simulink model "sistema_polo_polo"  (R2016a)
settings: Solver=ode45  SolverMode=SingleTasking  StartTime=0  StopTime=1.58  FixedStep=Ts_Power  RelTol=1e-3  AbsTol=1e-2
InitFcn:
  | Fnom = 50;        % Hz
  | 
  | Fc = 27*Fnom;   % (Hz)
  | Ts_Power = 1/(Fc*100);
  | Ts_Control = Ts_Power*10;
values from neighbouring files (symbols this model uses):
  L = 5    [obtencaodados.m]
undefined symbols (not defined in the file or in its folder): D1, Delta, DiscIntNeverNeededParam, magnitude
libraries: powerlib_meascontrol x56, powerlib x52
(part 4 of 4)

== system sistema_polo_polo/VSC Controller Station 2/Discrete VSC Controller /Signal Calculations/Filter_Bus_Voltage ==
  note: Filter Bus Voltage Calculation
  Uf_AB : Inport
  Math Function : Math  Operator=magnitude^2  SaturateOnIntegerOverflow=on
  Math Function1 : Math  Operator=sqrt  SaturateOnIntegerOverflow=on
  Sum : Sum  Inputs=+  SaturateOnIntegerOverflow=on
  Uf_meas : Outport
  wires:
  Math Function1/1 -> Uf_meas/1
  Sum/1 -> Math Function1/1
  Math Function/1 -> Sum/1
  Uf_AB/1 -> Math Function/1

== system sistema_polo_polo/VSC Controller Station 2/Discrete VSC Controller /Signal Calculations/Modulation_Index ==
  note: Modulation Index Calculation
  Vref_lim_AB : Inport
  Udc_meas : Inport  Port=2
  Gain1 : Gain  Gain=k_pu2nom_Vdc  SaturateOnIntegerOverflow=on  OutDataTypeStr=Inherit: Same as input  ParamDataTypeStr=Inherit: Same as input
  MAX:10 MIN: 0 : Saturate  UpperLimit=10  LowerLimit=0
  Math Function1 : Math  Operator=magnitude^2  SaturateOnIntegerOverflow=on
  Math Function2 : Math  Operator=sqrt  SaturateOnIntegerOverflow=on
  Product : Product  Inputs=*/  SaturateOnIntegerOverflow=on  OutDataTypeStr=Inherit: Same as first input
  Saturation : Saturate  UpperLimit=1e6  LowerLimit=1e-6
  Sum : Sum  Inputs=+  SaturateOnIntegerOverflow=on
  Mod_index : Outport
  wires:
  Gain1/1 -> Saturation/1
  MAX:10 MIN: 0/1 -> Mod_index/1
  Saturation/1 -> Product/2
  Product/1 -> MAX:10 MIN: 0/1
  Udc_meas/1 -> Gain1/1
  Sum/1 -> Math Function2/1
  Math Function1/1 -> Sum/1
  Math Function2/1 -> Product/1
  Vref_lim_AB/1 -> Math Function1/1

== system sistema_polo_polo/VSC Controller Station 2/Discrete VSC Controller /Signal Calculations/PCC_Voltage ==
  note: Active Power Calculation
  U_AB : Inport
  Math Function : Math  Operator=magnitude^2  SaturateOnIntegerOverflow=on
  Math Function1 : Math  Operator=sqrt  SaturateOnIntegerOverflow=on
  Sum : Sum  Inputs=+  SaturateOnIntegerOverflow=on
  Upcc : Outport
  wires:
  U_AB/1 -> Math Function/1
  Math Function/1 -> Sum/1
  Sum/1 -> Math Function1/1
  Math Function1/1 -> Upcc/1

== system sistema_polo_polo/VSC Controller Station 2/Discrete VSC Controller /Signal Calculations/Reactive_Power ==
  note: Reactive Power Calculation
  U_AB : Inport
  I_AB : Inport  Port=2
  Demux : Demux  Outputs=2
  Demux1 : Demux  Outputs=2
  Product : Product  SaturateOnIntegerOverflow=on  OutDataTypeStr=Inherit: Same as first input
  Product1 : Product  SaturateOnIntegerOverflow=on  OutDataTypeStr=Inherit: Same as first input
  Sum : Sum  Inputs=+-  SaturateOnIntegerOverflow=on
  Qpcc : Outport
  wires:
  Sum/1 -> Qpcc/1
  Product1/1 -> Sum/2
  Product/1 -> Sum/1
  I_AB/1 -> Demux1/1
  U_AB/1 -> Demux/1
  Demux/2 -> Product/2
  Demux1/1 -> Product/1
  Demux/1 -> Product1/1
  Demux1/2 -> Product1/2

== system sistema_polo_polo/VSC Controller Station 1/Discrete VSC Controller /Clark Transformations/CLARK  with Rotating reference/CLARK ==
  note: CLARK transformation
  abc : Inport
  Enable (held) : EnablePort  PropagateVarSize=During execution
  abc to Alpha-Beta-Zero : powerlib_meascontrol/Transformations/abc to Alpha-Beta-Zero
  AB0 : Outport
  wires:
  abc to Alpha-Beta-Zero/1 -> AB0/1
  abc/1 -> abc to Alpha-Beta-Zero/1

== system sistema_polo_polo/VSC Controller Station 1/Discrete VSC Controller /Clark Transformations/CLARK  with Rotating reference/CLARK_lag ==
  note: CLARK transformation - YD1
  abc : Inport
  Enable : EnablePort  PropagateVarSize=During execution
  Fcn1 : Fcn  Expr=(-u[1] - u[3] + 2*u[2] )/3
  Fcn2 : Fcn  Expr=(u[1]-u[3])/sqrt(3)
  Fcn3 : Fcn  Expr=0
  Mux : Mux  Inputs=3
  AB0 : Outport
  wires:
  Fcn2/1 -> Mux/1
  abc/1 -> Fcn1/1, Fcn3/1, Fcn2/1
  Fcn1/1 -> Mux/2
  Fcn3/1 -> Mux/3
  Mux/1 -> AB0/1

== system sistema_polo_polo/VSC Controller Station 1/Discrete VSC Controller /Clark Transformations/CLARK  with Rotating reference/CLARK_lead ==
  note: CLARK transformation - YD11
  abc : Inport
  Enable : EnablePort  PropagateVarSize=During execution
  Fcn1 : Fcn  Expr=(u[1] + u[2] - 2*u[3] )/3
  Fcn2 : Fcn  Expr=(u[1]-u[2])/sqrt(3)
  Fcn3 : Fcn  Expr=0
  Mux : Mux  Inputs=3
  AB0 : Outport
  wires:
  Mux/1 -> AB0/1
  Fcn3/1 -> Mux/3
  Fcn1/1 -> Mux/2
  abc/1 -> Fcn2/1, Fcn3/1, Fcn1/1
  Fcn2/1 -> Mux/1

== system sistema_polo_polo/VSC Controller Station 1/Discrete VSC Controller /Clark Transformations/CLARK  with Rotating reference1/CLARK ==
  note: CLARK transformation
  abc : Inport
  Enable (held) : EnablePort  PropagateVarSize=During execution
  abc to Alpha-Beta-Zero : powerlib_meascontrol/Transformations/abc to Alpha-Beta-Zero
  AB0 : Outport
  wires:
  abc to Alpha-Beta-Zero/1 -> AB0/1
  abc/1 -> abc to Alpha-Beta-Zero/1

== system sistema_polo_polo/VSC Controller Station 1/Discrete VSC Controller /Clark Transformations/CLARK  with Rotating reference1/CLARK_lag ==
  note: CLARK transformation - YD1
  abc : Inport
  Enable : EnablePort  PropagateVarSize=During execution
  Fcn1 : Fcn  Expr=(-u[1] - u[3] + 2*u[2] )/3
  Fcn2 : Fcn  Expr=(u[1]-u[3])/sqrt(3)
  Fcn3 : Fcn  Expr=0
  Mux : Mux  Inputs=3
  AB0 : Outport
  wires:
  Fcn2/1 -> Mux/1
  abc/1 -> Fcn1/1, Fcn3/1, Fcn2/1
  Fcn1/1 -> Mux/2
  Fcn3/1 -> Mux/3
  Mux/1 -> AB0/1

== system sistema_polo_polo/VSC Controller Station 1/Discrete VSC Controller /Clark Transformations/CLARK  with Rotating reference1/CLARK_lead ==
  note: CLARK transformation - YD11
  abc : Inport
  Enable : EnablePort  PropagateVarSize=During execution
  Fcn1 : Fcn  Expr=(u[1] + u[2] - 2*u[3] )/3
  Fcn2 : Fcn  Expr=(u[1]-u[2])/sqrt(3)
  Fcn3 : Fcn  Expr=0
  Mux : Mux  Inputs=3
  AB0 : Outport
  wires:
  Mux/1 -> AB0/1
  Fcn3/1 -> Mux/3
  Fcn1/1 -> Mux/2
  abc/1 -> Fcn2/1, Fcn3/1, Fcn1/1
  Fcn2/1 -> Mux/1

== system sistema_polo_polo/VSC Controller Station 1/Discrete VSC Controller /DC Voltage Balance Control/Regulator/PI_regulator (type 2) ==
  note: Regulator PI
      | (Type 2)
  Ord : Inport
  Meas : Inport  Port=2
  Add : Sum
  Add1 : Sum
  Discrete-Time Integrator : DiscreteIntegrator  IntegratorMethod=Integration: Trapezoidal  gainval=Ki  InitialCondition=i_ic  SampleTime=Ts  LimitOutput=on  UpperSaturationLimit=max_i  LowerSaturationLimit=min_i  ICPrevOutput=DiscIntNeverNeededParam  ICPrevScaledInput=DiscIntNeverNeededParam
      settings: AttributesFormatString=Gain=%<gainval>\nMin=%<LowerSaturationLimit>\nMax=%<UpperSaturationLimit>
  Kf : Gain  Gain=Kf
      settings: AttributesFormatString=Gain=%<Gain>
  Kp : Gain  Gain=Kp
      settings: AttributesFormatString=Gain=%<Gain>
  Saturation : Saturate  UpperLimit=max_out  LowerLimit=min_out
      settings: AttributesFormatString=Min=%<LowerLimit>\nMax=%<UpperLimit>
  Subtract : Sum  Inputs=+-
  Sum2 : Sum  Inputs=|+-  SaturateOnIntegerOverflow=on
  Unit Delay : UnitDelay  SampleTime=Ts_Control
      settings: AttributesFormatString=IC=%<InitialCondition>
  Out : Outport
  wires:
  Kp/1 -> Add1/1
  Sum2/1 -> Kf/1
  Subtract/1 -> Add/1, Kp/1
  Saturation/1 -> Sum2/1, Out/1
  Unit Delay/1 -> Add/2
  Add/1 -> Discrete-Time Integrator/1
  Ord/1 -> Subtract/1
  Kf/1 -> Unit Delay/1
  Add1/1 -> Saturation/1, Sum2/2
  Discrete-Time Integrator/1 -> Add1/2
  Meas/1 -> Subtract/2

== system sistema_polo_polo/VSC Controller Station 1/Discrete VSC Controller /Inner Current Loop/AC_Current_Control/PI_regulator 1 ==
  note: Regulator PI
      | (Type 2)
  Ord : Inport
  Meas : Inport  Port=2
  Add : Sum
  Add1 : Sum
  Discrete-Time Integrator : DiscreteIntegrator  IntegratorMethod=Integration: Trapezoidal  gainval=Ki  InitialCondition=i_ic  SampleTime=Ts  LimitOutput=on  UpperSaturationLimit=max_i  LowerSaturationLimit=min_i  ICPrevOutput=DiscIntNeverNeededParam  ICPrevScaledInput=DiscIntNeverNeededParam
      settings: AttributesFormatString=Gain=%<gainval>\nMin=%<LowerSaturationLimit>\nMax=%<UpperSaturationLimit>
  Kf : Gain  Gain=Kf
      settings: AttributesFormatString=Gain=%<Gain>
  Kp : Gain  Gain=Kp
      settings: AttributesFormatString=Gain=%<Gain>
  Saturation : Saturate  UpperLimit=max_out  LowerLimit=min_out
      settings: AttributesFormatString=Min=%<LowerLimit>\nMax=%<UpperLimit>
  Subtract : Sum  Inputs=+-
  Sum2 : Sum  Inputs=|+-  SaturateOnIntegerOverflow=on
  Unit Delay : UnitDelay  SampleTime=Ts_Control
      settings: AttributesFormatString=IC=%<InitialCondition>
  Out : Outport
  wires:
  Kp/1 -> Add1/1
  Sum2/1 -> Kf/1
  Subtract/1 -> Add/1, Kp/1
  Saturation/1 -> Sum2/1, Out/1
  Unit Delay/1 -> Add/2
  Add/1 -> Discrete-Time Integrator/1
  Ord/1 -> Subtract/1
  Kf/1 -> Unit Delay/1
  Add1/1 -> Saturation/1, Sum2/2
  Discrete-Time Integrator/1 -> Add1/2
  Meas/1 -> Subtract/2

== system sistema_polo_polo/VSC Controller Station 1/Discrete VSC Controller /Inner Current Loop/AC_Current_Control/PI_regulator 2 ==
  note: Regulator PI
      | (Type 2)
  Ord : Inport
  Meas : Inport  Port=2
  Add : Sum
  Add1 : Sum
  Discrete-Time Integrator : DiscreteIntegrator  IntegratorMethod=Integration: Trapezoidal  gainval=Ki  InitialCondition=i_ic  SampleTime=Ts  LimitOutput=on  UpperSaturationLimit=max_i  LowerSaturationLimit=min_i  ICPrevOutput=DiscIntNeverNeededParam  ICPrevScaledInput=DiscIntNeverNeededParam
      settings: AttributesFormatString=Gain=%<gainval>\nMin=%<LowerSaturationLimit>\nMax=%<UpperSaturationLimit>
  Kf : Gain  Gain=Kf
      settings: AttributesFormatString=Gain=%<Gain>
  Kp : Gain  Gain=Kp
      settings: AttributesFormatString=Gain=%<Gain>
  Saturation : Saturate  UpperLimit=max_out  LowerLimit=min_out
      settings: AttributesFormatString=Min=%<LowerLimit>\nMax=%<UpperLimit>
  Subtract : Sum  Inputs=+-
  Sum2 : Sum  Inputs=|+-  SaturateOnIntegerOverflow=on
  Unit Delay : UnitDelay  SampleTime=Ts_Control
      settings: AttributesFormatString=IC=%<InitialCondition>
  Out : Outport
  wires:
  Kp/1 -> Add1/1
  Sum2/1 -> Kf/1
  Subtract/1 -> Add/1, Kp/1
  Saturation/1 -> Sum2/1, Out/1
  Unit Delay/1 -> Add/2
  Add/1 -> Discrete-Time Integrator/1
  Ord/1 -> Subtract/1
  Kf/1 -> Unit Delay/1
  Add1/1 -> Saturation/1, Sum2/2
  Discrete-Time Integrator/1 -> Add1/2
  Meas/1 -> Subtract/2

== system sistema_polo_polo/VSC Controller Station 1/Discrete VSC Controller /Outer Active-Reactive Power and Voltage Loop/Active_Power_Control/DC Voltage Control Override ==
  note: Reset states when enabling
  note: Override Regulator
  note: Active when input (In) is outside its range [min_in, max_in] otherwise the output goes back to zero
  In : Inport
  Enable (reset) : EnablePort  StatesWhenEnabling=reset  PropagateVarSize=During execution
  Add : Sum
  Constant1 : Constant  Value=max_in
  Constant2 : Constant  Value=min_in
  Constant3 : Constant  Value=Kp
  Discrete-Time Integrator1 : DiscreteIntegrator  IntegratorMethod=Integration: Trapezoidal  gainval=Ki  InitialCondition=IC_i  SampleTime=Ts  LimitOutput=on  UpperSaturationLimit=0  LowerSaturationLimit=min_out_lim  ICPrevOutput=DiscIntNeverNeededParam  ICPrevScaledInput=DiscIntNeverNeededParam
      settings: AttributesFormatString=Gain=%<gainval>\nMin=%<LowerSaturationLimit>\nMax=%<UpperSaturationLimit>
  Discrete-Time Integrator2 : DiscreteIntegrator  IntegratorMethod=Integration: Trapezoidal  gainval=Ki  InitialCondition=IC_i  SampleTime=Ts  LimitOutput=on  UpperSaturationLimit=max_out_lim  LowerSaturationLimit=0  ICPrevOutput=DiscIntNeverNeededParam  ICPrevScaledInput=DiscIntNeverNeededParam
      settings: AttributesFormatString=Gain=%<gainval>\nMin=%<LowerSaturationLimit>\nMax=%<UpperSaturationLimit>
  Product : Product  RndMeth=Zero
  Saturation : Saturate  UpperLimit=0  LowerLimit=min_out_lim
      settings: AttributesFormatString=Min=%<LowerLimit>\nMax=%<UpperLimit>
  Saturation1 : Saturate  UpperLimit=max_out_lim  LowerLimit=0
      settings: AttributesFormatString=Min=%<LowerLimit>\nMax=%<UpperLimit>
  Saturation2 : Saturate  UpperLimit=max_out_lim  LowerLimit=min_out_lim
      settings: AttributesFormatString=Min=%<LowerLimit>\nMax=%<UpperLimit>
  Subtract : Sum  Inputs=+-
  Subtract1 : Sum  Inputs=-+
  Sum2 : Sum  Inputs=+++  SaturateOnIntegerOverflow=on
  Out : Outport
  wires:
  Constant2/1 -> Subtract1/2
  Constant1/1 -> Subtract/1
  Discrete-Time Integrator2/1 -> Sum2/3  "positive"
  Discrete-Time Integrator1/1 -> Sum2/2  "negative"
  Product/1 -> Sum2/1
  Saturation1/1 -> Add/2
  Saturation/1 -> Add/1
  Add/1 -> Product/2
  Constant3/1 -> Product/1
  In/1 -> Subtract1/1, Subtract/2
  Subtract/1 -> Discrete-Time Integrator1/1, Saturation/1
  Subtract1/1 -> Saturation1/1, Discrete-Time Integrator2/1
  Sum2/1 -> Saturation2/1
  Saturation2/1 -> Out/1

== system sistema_polo_polo/VSC Controller Station 1/Discrete VSC Controller /Outer Active-Reactive Power and Voltage Loop/Active_Power_Control/Freeze_integrator ==
  note: Low AC voltage level
  note: Freeze Integrator
  U_meas : Inport
  Constant8 : Constant  Value=V_level_apc
  Relational Operator : RelationalOperator  Operator=<=
  Freeze : Outport
  wires:
  Constant8/1 -> Relational Operator/2
  Relational Operator/1 -> Freeze/1
  U_meas/1 -> Relational Operator/1

== system sistema_polo_polo/VSC Controller Station 1/Discrete VSC Controller /Outer Active-Reactive Power and Voltage Loop/Active_Power_Control/Int_regulator (type 1) ==
  note: Reset states when enabling
  note: Integral Regulator
      | (Type 1)
  Ord : Inport
  Meas : Inport  Port=2
  freeze : Inport  Port=3
  Enable (Reset) : EnablePort  StatesWhenEnabling=reset  PropagateVarSize=During execution
  Add : Sum
  Add1 : Sum
  Constant7 : Constant  Value=0.0
  Discrete-Time Integrator : DiscreteIntegrator  IntegratorMethod=Integration: Trapezoidal  gainval=Ki  InitialCondition=IC_i  SampleTime=Ts  LimitOutput=on  UpperSaturationLimit=max_i  LowerSaturationLimit=min_i  ICPrevOutput=DiscIntNeverNeededParam  ICPrevScaledInput=DiscIntNeverNeededParam
      settings: AttributesFormatString=Gain=%<gainval>\nMin=%<LowerSaturationLimit>\nMax=%<UpperSaturationLimit>
  Kf : Gain  Gain=Kf
      settings: AttributesFormatString=Gain=%<Gain>
  Saturation : Saturate  UpperLimit=max_out  LowerLimit=min_out
      settings: AttributesFormatString=Min=%<LowerLimit>\nMax=%<UpperLimit>
  Subtract : Sum  Inputs=+-
  Sum2 : Sum  Inputs=|+-  SaturateOnIntegerOverflow=on
  Switch : Switch  Criteria=u2 > Threshold  SaturateOnIntegerOverflow=on
  Unit Delay : UnitDelay  SampleTime=Ts_Control
      settings: AttributesFormatString=IC=%<InitialCondition>
  Out : Outport
  wires:
  Kf/1 -> Unit Delay/1
  Subtract/1 -> Switch/3
  Meas/1 -> Subtract/2
  Switch/1 -> Add/1
  Constant7/1 -> Switch/1
  freeze/1 -> Switch/2
  Discrete-Time Integrator/1 -> Add1/2
  Add1/1 -> Sum2/2, Saturation/1
  Sum2/1 -> Kf/1
  Ord/1 -> Subtract/1, Add1/1
  Add/1 -> Discrete-Time Integrator/1
  Unit Delay/1 -> Add/2
  Saturation/1 -> Sum2/1, Out/1

== system sistema_polo_polo/VSC Controller Station 1/Discrete VSC Controller /Outer Active-Reactive Power and Voltage Loop/Active_Power_Control/Ramping ==
  note: Output is reset to zero when the ramp is not enabled
  note: Ramping
  enable_ramp : Inport
  Pref : Inport  Port=2
  Constant12 : Constant  Value=Ramp_apc
  Logical Operator7 : Logic  Operator=NOT  AllPortsSameDT=off
  Rate Limiter with external rates & reset (discrete) IC:0 : Subsystem  mask(Rate of Change Limiter){ic=0, st=Ts_Control}
      mask prompts: ic "Initial condition (pu):"; st "Sample time (s):"
      mask help: Limit rising and falling rates of signal. When the input (R) is true the output is reset to the input (In). Rates are in p.u./s for up and -p.u./s for down.
      mask Display: disp('                Rate\n               Limiter')
  Switch : Switch  Criteria=u2 > Threshold  SaturateOnIntegerOverflow=on
  zero : Constant  Value=0.0
  Pref_ramp : Outport
  wires:
  Logical Operator7/1 -> Rate Limiter with external rates & reset (discrete) IC:0/4(R)
  Switch/1 -> Rate Limiter with external rates & reset (discrete) IC:0/1(In)
  zero/1 -> Switch/3
  Pref/1 -> Switch/1
  enable_ramp/1 -> Logical Operator7/1, Switch/2
  Constant12/1 -> Rate Limiter with external rates & reset (discrete) IC:0/3(down_rate), Rate Limiter with external rates & reset (discrete) IC:0/2(up_rate)
  Rate Limiter with external rates & reset (discrete) IC:0/1(" ") -> Pref_ramp/1

== system sistema_polo_polo/VSC Controller Station 1/Discrete VSC Controller /Outer Active-Reactive Power and Voltage Loop/Current_Reference_Limitation/Double click here for  info ==
  note: Power System Simulation laboratory (IREQ)
  note: Current Reference Limitation
  note: The subsystem limits the amplitude of phase current of the fundamental component to the rated current
      | of the converter.
  note: Power Control Mode
  note: DC Voltage Control Mode
  note: In power control mode, equal scaling is applied to the active and reactive power reference when a limit is imposed.
  note: In DC voltage control mode, higher priority is given to the active power when a limit is imposed.

== system sistema_polo_polo/VSC Controller Station 1/Discrete VSC Controller /Outer Active-Reactive Power and Voltage Loop/DC_Voltage_Control/PI_regulator (type 2) ==
  note: Regulator PI
      | (Type 2)
  Ord : Inport
  Meas : Inport  Port=2
  Add : Sum
  Add1 : Sum
  Discrete-Time Integrator : DiscreteIntegrator  IntegratorMethod=Integration: Trapezoidal  gainval=Ki  InitialCondition=i_ic  SampleTime=Ts  LimitOutput=on  UpperSaturationLimit=max_i  LowerSaturationLimit=min_i  ICPrevOutput=DiscIntNeverNeededParam  ICPrevScaledInput=DiscIntNeverNeededParam
      settings: AttributesFormatString=Gain=%<gainval>\nMin=%<LowerSaturationLimit>\nMax=%<UpperSaturationLimit>
  Kf : Gain  Gain=Kf
      settings: AttributesFormatString=Gain=%<Gain>
  Kp : Gain  Gain=Kp
      settings: AttributesFormatString=Gain=%<Gain>
  Saturation : Saturate  UpperLimit=max_out  LowerLimit=min_out
      settings: AttributesFormatString=Min=%<LowerLimit>\nMax=%<UpperLimit>
  Subtract : Sum  Inputs=+-
  Sum2 : Sum  Inputs=|+-  SaturateOnIntegerOverflow=on
  Unit Delay : UnitDelay  SampleTime=Ts_Control
      settings: AttributesFormatString=IC=%<InitialCondition>
  Out : Outport
  wires:
  Kp/1 -> Add1/1
  Sum2/1 -> Kf/1
  Subtract/1 -> Add/1, Kp/1
  Saturation/1 -> Sum2/1, Out/1
  Unit Delay/1 -> Add/2
  Add/1 -> Discrete-Time Integrator/1
  Ord/1 -> Subtract/1
  Kf/1 -> Unit Delay/1
  Add1/1 -> Saturation/1, Sum2/2
  Discrete-Time Integrator/1 -> Add1/2
  Meas/1 -> Subtract/2

== system sistema_polo_polo/VSC Controller Station 1/Discrete VSC Controller /Outer Active-Reactive Power and Voltage Loop/Reactive_Power_Control/AC Voltage Control Override  ==
  note: Reset states when enabling
  note: Override Regulator
  note: Active when input (In) is outside its range [min_in, max_in] otherwise the output goes back to zero
  In : Inport
  Enable (reset) : EnablePort  StatesWhenEnabling=reset  PropagateVarSize=During execution
  Add : Sum
  Constant1 : Constant  Value=max_in
  Constant2 : Constant  Value=min_in
  Constant3 : Constant  Value=Kp
  Discrete-Time Integrator1 : DiscreteIntegrator  IntegratorMethod=Integration: Trapezoidal  gainval=Ki  InitialCondition=IC_i  SampleTime=Ts  LimitOutput=on  UpperSaturationLimit=0  LowerSaturationLimit=min_out_lim  ICPrevOutput=DiscIntNeverNeededParam  ICPrevScaledInput=DiscIntNeverNeededParam
      settings: AttributesFormatString=Gain=%<gainval>\nMin=%<LowerSaturationLimit>\nMax=%<UpperSaturationLimit>
  Discrete-Time Integrator2 : DiscreteIntegrator  IntegratorMethod=Integration: Trapezoidal  gainval=Ki  InitialCondition=IC_i  SampleTime=Ts  LimitOutput=on  UpperSaturationLimit=max_out_lim  LowerSaturationLimit=0  ICPrevOutput=DiscIntNeverNeededParam  ICPrevScaledInput=DiscIntNeverNeededParam
      settings: AttributesFormatString=Gain=%<gainval>\nMin=%<LowerSaturationLimit>\nMax=%<UpperSaturationLimit>
  Product : Product  RndMeth=Zero
  Saturation : Saturate  UpperLimit=0  LowerLimit=min_out_lim
      settings: AttributesFormatString=Min=%<LowerLimit>\nMax=%<UpperLimit>
  Saturation1 : Saturate  UpperLimit=max_out_lim  LowerLimit=0
      settings: AttributesFormatString=Min=%<LowerLimit>\nMax=%<UpperLimit>
  Saturation2 : Saturate  UpperLimit=max_out_lim  LowerLimit=min_out_lim
      settings: AttributesFormatString=Min=%<LowerLimit>\nMax=%<UpperLimit>
  Subtract : Sum  Inputs=+-
  Subtract1 : Sum  Inputs=-+
  Sum2 : Sum  Inputs=+++  SaturateOnIntegerOverflow=on
  Out : Outport
  wires:
  Constant2/1 -> Subtract1/2
  Constant1/1 -> Subtract/1
  Discrete-Time Integrator2/1 -> Sum2/3  "positive"
  Discrete-Time Integrator1/1 -> Sum2/2  "negative"
  Product/1 -> Sum2/1
  Saturation1/1 -> Add/2
  Saturation/1 -> Add/1
  Add/1 -> Product/2
  Constant3/1 -> Product/1
  In/1 -> Subtract1/1, Subtract/2
  Subtract/1 -> Discrete-Time Integrator1/1, Saturation/1
  Subtract1/1 -> Saturation1/1, Discrete-Time Integrator2/1
  Sum2/1 -> Saturation2/1
  Saturation2/1 -> Out/1

== system sistema_polo_polo/VSC Controller Station 1/Discrete VSC Controller /Outer Active-Reactive Power and Voltage Loop/Reactive_Power_Control/Freeze_integrator ==
  note: Freeze Integrator
  note: Low AC voltage level
  U_meas : Inport
  Constant8 : Constant  Value=V_level_rpc
  Relational Operator : RelationalOperator  Operator=<=
  Freeze : Outport
  wires:
  U_meas/1 -> Relational Operator/1
  Relational Operator/1 -> Freeze/1
  Constant8/1 -> Relational Operator/2

== system sistema_polo_polo/VSC Controller Station 1/Discrete VSC Controller /Outer Active-Reactive Power and Voltage Loop/Reactive_Power_Control/Int_regulator (type 1) ==
  note: Reset states when enabling
  note: Integral Regulator
      | (Type 1)
  Ord : Inport
  Meas : Inport  Port=2
  freeze : Inport  Port=3
  Enable (Reset) : EnablePort  StatesWhenEnabling=reset  PropagateVarSize=During execution
  Add : Sum
  Add1 : Sum
  Constant7 : Constant  Value=0.0
  Discrete-Time Integrator : DiscreteIntegrator  IntegratorMethod=Integration: Trapezoidal  gainval=Ki  InitialCondition=IC_i  SampleTime=Ts  LimitOutput=on  UpperSaturationLimit=max_i  LowerSaturationLimit=min_i  ICPrevOutput=DiscIntNeverNeededParam  ICPrevScaledInput=DiscIntNeverNeededParam
      settings: AttributesFormatString=Gain=%<gainval>\nMin=%<LowerSaturationLimit>\nMax=%<UpperSaturationLimit>
  Kf : Gain  Gain=Kf
      settings: AttributesFormatString=Gain=%<Gain>
  Saturation : Saturate  UpperLimit=max_out  LowerLimit=min_out
      settings: AttributesFormatString=Min=%<LowerLimit>\nMax=%<UpperLimit>
  Subtract : Sum  Inputs=+-
  Sum2 : Sum  Inputs=|+-  SaturateOnIntegerOverflow=on
  Switch : Switch  Criteria=u2 > Threshold  SaturateOnIntegerOverflow=on
  Unit Delay : UnitDelay  SampleTime=Ts_Control
      settings: AttributesFormatString=IC=%<InitialCondition>
  Out : Outport
  wires:
  Kf/1 -> Unit Delay/1
  Subtract/1 -> Switch/3
  Meas/1 -> Subtract/2
  Switch/1 -> Add/1
  Constant7/1 -> Switch/1
  freeze/1 -> Switch/2
  Discrete-Time Integrator/1 -> Add1/2
  Add1/1 -> Sum2/2, Saturation/1
  Sum2/1 -> Kf/1
  Ord/1 -> Subtract/1, Add1/1
  Add/1 -> Discrete-Time Integrator/1
  Unit Delay/1 -> Add/2
  Saturation/1 -> Sum2/1, Out/1

== system sistema_polo_polo/VSC Controller Station 2/Discrete VSC Controller /Clark Transformations/CLARK  with Rotating reference/CLARK ==
  note: CLARK transformation
  abc : Inport
  Enable (held) : EnablePort  PropagateVarSize=During execution
  abc to Alpha-Beta-Zero : powerlib_meascontrol/Transformations/abc to Alpha-Beta-Zero
  AB0 : Outport
  wires:
  abc to Alpha-Beta-Zero/1 -> AB0/1
  abc/1 -> abc to Alpha-Beta-Zero/1

== system sistema_polo_polo/VSC Controller Station 2/Discrete VSC Controller /Clark Transformations/CLARK  with Rotating reference/CLARK_lag ==
  note: CLARK transformation - YD1
  abc : Inport
  Enable : EnablePort  PropagateVarSize=During execution
  Fcn1 : Fcn  Expr=(-u[1] - u[3] + 2*u[2] )/3
  Fcn2 : Fcn  Expr=(u[1]-u[3])/sqrt(3)
  Fcn3 : Fcn  Expr=0
  Mux : Mux  Inputs=3
  AB0 : Outport
  wires:
  Fcn2/1 -> Mux/1
  abc/1 -> Fcn1/1, Fcn3/1, Fcn2/1
  Fcn1/1 -> Mux/2
  Fcn3/1 -> Mux/3
  Mux/1 -> AB0/1

== system sistema_polo_polo/VSC Controller Station 2/Discrete VSC Controller /Clark Transformations/CLARK  with Rotating reference/CLARK_lead ==
  note: CLARK transformation - YD11
  abc : Inport
  Enable : EnablePort  PropagateVarSize=During execution
  Fcn1 : Fcn  Expr=(u[1] + u[2] - 2*u[3] )/3
  Fcn2 : Fcn  Expr=(u[1]-u[2])/sqrt(3)
  Fcn3 : Fcn  Expr=0
  Mux : Mux  Inputs=3
  AB0 : Outport
  wires:
  Mux/1 -> AB0/1
  Fcn3/1 -> Mux/3
  Fcn1/1 -> Mux/2
  abc/1 -> Fcn2/1, Fcn3/1, Fcn1/1
  Fcn2/1 -> Mux/1

== system sistema_polo_polo/VSC Controller Station 2/Discrete VSC Controller /Clark Transformations/CLARK  with Rotating reference1/CLARK ==
  note: CLARK transformation
  abc : Inport
  Enable (held) : EnablePort  PropagateVarSize=During execution
  abc to Alpha-Beta-Zero : powerlib_meascontrol/Transformations/abc to Alpha-Beta-Zero
  AB0 : Outport
  wires:
  abc to Alpha-Beta-Zero/1 -> AB0/1
  abc/1 -> abc to Alpha-Beta-Zero/1

== system sistema_polo_polo/VSC Controller Station 2/Discrete VSC Controller /Clark Transformations/CLARK  with Rotating reference1/CLARK_lag ==
  note: CLARK transformation - YD1
  abc : Inport
  Enable : EnablePort  PropagateVarSize=During execution
  Fcn1 : Fcn  Expr=(-u[1] - u[3] + 2*u[2] )/3
  Fcn2 : Fcn  Expr=(u[1]-u[3])/sqrt(3)
  Fcn3 : Fcn  Expr=0
  Mux : Mux  Inputs=3
  AB0 : Outport
  wires:
  Fcn2/1 -> Mux/1
  abc/1 -> Fcn1/1, Fcn3/1, Fcn2/1
  Fcn1/1 -> Mux/2
  Fcn3/1 -> Mux/3
  Mux/1 -> AB0/1

== system sistema_polo_polo/VSC Controller Station 2/Discrete VSC Controller /Clark Transformations/CLARK  with Rotating reference1/CLARK_lead ==
  note: CLARK transformation - YD11
  abc : Inport
  Enable : EnablePort  PropagateVarSize=During execution
  Fcn1 : Fcn  Expr=(u[1] + u[2] - 2*u[3] )/3
  Fcn2 : Fcn  Expr=(u[1]-u[2])/sqrt(3)
  Fcn3 : Fcn  Expr=0
  Mux : Mux  Inputs=3
  AB0 : Outport
  wires:
  Mux/1 -> AB0/1
  Fcn3/1 -> Mux/3
  Fcn1/1 -> Mux/2
  abc/1 -> Fcn2/1, Fcn3/1, Fcn1/1
  Fcn2/1 -> Mux/1

== system sistema_polo_polo/VSC Controller Station 2/Discrete VSC Controller /DC Voltage Balance Control/Regulator/PI_regulator (type 2) ==
  note: Regulator PI
      | (Type 2)
  Ord : Inport
  Meas : Inport  Port=2
  Add : Sum
  Add1 : Sum
  Discrete-Time Integrator : DiscreteIntegrator  IntegratorMethod=Integration: Trapezoidal  gainval=Ki  InitialCondition=i_ic  SampleTime=Ts  LimitOutput=on  UpperSaturationLimit=max_i  LowerSaturationLimit=min_i  ICPrevOutput=DiscIntNeverNeededParam  ICPrevScaledInput=DiscIntNeverNeededParam
      settings: AttributesFormatString=Gain=%<gainval>\nMin=%<LowerSaturationLimit>\nMax=%<UpperSaturationLimit>
  Kf : Gain  Gain=Kf
      settings: AttributesFormatString=Gain=%<Gain>
  Kp : Gain  Gain=Kp
      settings: AttributesFormatString=Gain=%<Gain>
  Saturation : Saturate  UpperLimit=max_out  LowerLimit=min_out
      settings: AttributesFormatString=Min=%<LowerLimit>\nMax=%<UpperLimit>
  Subtract : Sum  Inputs=+-
  Sum2 : Sum  Inputs=|+-  SaturateOnIntegerOverflow=on
  Unit Delay : UnitDelay  SampleTime=Ts_Control
      settings: AttributesFormatString=IC=%<InitialCondition>
  Out : Outport
  wires:
  Kp/1 -> Add1/1
  Sum2/1 -> Kf/1
  Subtract/1 -> Add/1, Kp/1
  Saturation/1 -> Sum2/1, Out/1
  Unit Delay/1 -> Add/2
  Add/1 -> Discrete-Time Integrator/1
  Ord/1 -> Subtract/1
  Kf/1 -> Unit Delay/1
  Add1/1 -> Saturation/1, Sum2/2
  Discrete-Time Integrator/1 -> Add1/2
  Meas/1 -> Subtract/2

== system sistema_polo_polo/VSC Controller Station 2/Discrete VSC Controller /Inner Current Loop/AC_Current_Control/PI_regulator 1 ==
  note: Regulator PI
      | (Type 2)
  Ord : Inport
  Meas : Inport  Port=2
  Add : Sum
  Add1 : Sum
  Discrete-Time Integrator : DiscreteIntegrator  IntegratorMethod=Integration: Trapezoidal  gainval=Ki  InitialCondition=i_ic  SampleTime=Ts  LimitOutput=on  UpperSaturationLimit=max_i  LowerSaturationLimit=min_i  ICPrevOutput=DiscIntNeverNeededParam  ICPrevScaledInput=DiscIntNeverNeededParam
      settings: AttributesFormatString=Gain=%<gainval>\nMin=%<LowerSaturationLimit>\nMax=%<UpperSaturationLimit>
  Kf : Gain  Gain=Kf
      settings: AttributesFormatString=Gain=%<Gain>
  Kp : Gain  Gain=Kp
      settings: AttributesFormatString=Gain=%<Gain>
  Saturation : Saturate  UpperLimit=max_out  LowerLimit=min_out
      settings: AttributesFormatString=Min=%<LowerLimit>\nMax=%<UpperLimit>
  Subtract : Sum  Inputs=+-
  Sum2 : Sum  Inputs=|+-  SaturateOnIntegerOverflow=on
  Unit Delay : UnitDelay  SampleTime=Ts_Control
      settings: AttributesFormatString=IC=%<InitialCondition>
  Out : Outport
  wires:
  Kp/1 -> Add1/1
  Sum2/1 -> Kf/1
  Subtract/1 -> Add/1, Kp/1
  Saturation/1 -> Sum2/1, Out/1
  Unit Delay/1 -> Add/2
  Add/1 -> Discrete-Time Integrator/1
  Ord/1 -> Subtract/1
  Kf/1 -> Unit Delay/1
  Add1/1 -> Saturation/1, Sum2/2
  Discrete-Time Integrator/1 -> Add1/2
  Meas/1 -> Subtract/2

== system sistema_polo_polo/VSC Controller Station 2/Discrete VSC Controller /Inner Current Loop/AC_Current_Control/PI_regulator 2 ==
  note: Regulator PI
      | (Type 2)
  Ord : Inport
  Meas : Inport  Port=2
  Add : Sum
  Add1 : Sum
  Discrete-Time Integrator : DiscreteIntegrator  IntegratorMethod=Integration: Trapezoidal  gainval=Ki  InitialCondition=i_ic  SampleTime=Ts  LimitOutput=on  UpperSaturationLimit=max_i  LowerSaturationLimit=min_i  ICPrevOutput=DiscIntNeverNeededParam  ICPrevScaledInput=DiscIntNeverNeededParam
      settings: AttributesFormatString=Gain=%<gainval>\nMin=%<LowerSaturationLimit>\nMax=%<UpperSaturationLimit>
  Kf : Gain  Gain=Kf
      settings: AttributesFormatString=Gain=%<Gain>
  Kp : Gain  Gain=Kp
      settings: AttributesFormatString=Gain=%<Gain>
  Saturation : Saturate  UpperLimit=max_out  LowerLimit=min_out
      settings: AttributesFormatString=Min=%<LowerLimit>\nMax=%<UpperLimit>
  Subtract : Sum  Inputs=+-
  Sum2 : Sum  Inputs=|+-  SaturateOnIntegerOverflow=on
  Unit Delay : UnitDelay  SampleTime=Ts_Control
      settings: AttributesFormatString=IC=%<InitialCondition>
  Out : Outport
  wires:
  Kp/1 -> Add1/1
  Sum2/1 -> Kf/1
  Subtract/1 -> Add/1, Kp/1
  Saturation/1 -> Sum2/1, Out/1
  Unit Delay/1 -> Add/2
  Add/1 -> Discrete-Time Integrator/1
  Ord/1 -> Subtract/1
  Kf/1 -> Unit Delay/1
  Add1/1 -> Saturation/1, Sum2/2
  Discrete-Time Integrator/1 -> Add1/2
  Meas/1 -> Subtract/2

== system sistema_polo_polo/VSC Controller Station 2/Discrete VSC Controller /Outer Active-Reactive Power and Voltage Loop/Active_Power_Control/DC Voltage Control Override ==
  note: Reset states when enabling
  note: Override Regulator
  note: Active when input (In) is outside its range [min_in, max_in] otherwise the output goes back to zero
  In : Inport
  Enable (reset) : EnablePort  StatesWhenEnabling=reset  PropagateVarSize=During execution
  Add : Sum
  Constant1 : Constant  Value=max_in
  Constant2 : Constant  Value=min_in
  Constant3 : Constant  Value=Kp
  Discrete-Time Integrator1 : DiscreteIntegrator  IntegratorMethod=Integration: Trapezoidal  gainval=Ki  InitialCondition=IC_i  SampleTime=Ts  LimitOutput=on  UpperSaturationLimit=0  LowerSaturationLimit=min_out_lim  ICPrevOutput=DiscIntNeverNeededParam  ICPrevScaledInput=DiscIntNeverNeededParam
      settings: AttributesFormatString=Gain=%<gainval>\nMin=%<LowerSaturationLimit>\nMax=%<UpperSaturationLimit>
  Discrete-Time Integrator2 : DiscreteIntegrator  IntegratorMethod=Integration: Trapezoidal  gainval=Ki  InitialCondition=IC_i  SampleTime=Ts  LimitOutput=on  UpperSaturationLimit=max_out_lim  LowerSaturationLimit=0  ICPrevOutput=DiscIntNeverNeededParam  ICPrevScaledInput=DiscIntNeverNeededParam
      settings: AttributesFormatString=Gain=%<gainval>\nMin=%<LowerSaturationLimit>\nMax=%<UpperSaturationLimit>
  Product : Product  RndMeth=Zero
  Saturation : Saturate  UpperLimit=0  LowerLimit=min_out_lim
      settings: AttributesFormatString=Min=%<LowerLimit>\nMax=%<UpperLimit>
  Saturation1 : Saturate  UpperLimit=max_out_lim  LowerLimit=0
      settings: AttributesFormatString=Min=%<LowerLimit>\nMax=%<UpperLimit>
  Saturation2 : Saturate  UpperLimit=max_out_lim  LowerLimit=min_out_lim
      settings: AttributesFormatString=Min=%<LowerLimit>\nMax=%<UpperLimit>
  Subtract : Sum  Inputs=+-
  Subtract1 : Sum  Inputs=-+
  Sum2 : Sum  Inputs=+++  SaturateOnIntegerOverflow=on
  Out : Outport
  wires:
  Constant2/1 -> Subtract1/2
  Constant1/1 -> Subtract/1
  Discrete-Time Integrator2/1 -> Sum2/3  "positive"
  Discrete-Time Integrator1/1 -> Sum2/2  "negative"
  Product/1 -> Sum2/1
  Saturation1/1 -> Add/2
  Saturation/1 -> Add/1
  Add/1 -> Product/2
  Constant3/1 -> Product/1
  In/1 -> Subtract1/1, Subtract/2
  Subtract/1 -> Discrete-Time Integrator1/1, Saturation/1
  Subtract1/1 -> Saturation1/1, Discrete-Time Integrator2/1
  Sum2/1 -> Saturation2/1
  Saturation2/1 -> Out/1

== system sistema_polo_polo/VSC Controller Station 2/Discrete VSC Controller /Outer Active-Reactive Power and Voltage Loop/Active_Power_Control/Freeze_integrator ==
  note: Low AC voltage level
  note: Freeze Integrator
  U_meas : Inport
  Constant8 : Constant  Value=V_level_apc
  Relational Operator : RelationalOperator  Operator=<=
  Freeze : Outport
  wires:
  Constant8/1 -> Relational Operator/2
  Relational Operator/1 -> Freeze/1
  U_meas/1 -> Relational Operator/1

== system sistema_polo_polo/VSC Controller Station 2/Discrete VSC Controller /Outer Active-Reactive Power and Voltage Loop/Active_Power_Control/Int_regulator (type 1) ==
  note: Reset states when enabling
  note: Integral Regulator
      | (Type 1)
  Ord : Inport
  Meas : Inport  Port=2
  freeze : Inport  Port=3
  Enable (Reset) : EnablePort  StatesWhenEnabling=reset  PropagateVarSize=During execution
  Add : Sum
  Add1 : Sum
  Constant7 : Constant  Value=0.0
  Discrete-Time Integrator : DiscreteIntegrator  IntegratorMethod=Integration: Trapezoidal  gainval=Ki  InitialCondition=IC_i  SampleTime=Ts  LimitOutput=on  UpperSaturationLimit=max_i  LowerSaturationLimit=min_i  ICPrevOutput=DiscIntNeverNeededParam  ICPrevScaledInput=DiscIntNeverNeededParam
      settings: AttributesFormatString=Gain=%<gainval>\nMin=%<LowerSaturationLimit>\nMax=%<UpperSaturationLimit>
  Kf : Gain  Gain=Kf
      settings: AttributesFormatString=Gain=%<Gain>
  Saturation : Saturate  UpperLimit=max_out  LowerLimit=min_out
      settings: AttributesFormatString=Min=%<LowerLimit>\nMax=%<UpperLimit>
  Subtract : Sum  Inputs=+-
  Sum2 : Sum  Inputs=|+-  SaturateOnIntegerOverflow=on
  Switch : Switch  Criteria=u2 > Threshold  SaturateOnIntegerOverflow=on
  Unit Delay : UnitDelay  SampleTime=Ts_Control
      settings: AttributesFormatString=IC=%<InitialCondition>
  Out : Outport
  wires:
  Kf/1 -> Unit Delay/1
  Subtract/1 -> Switch/3
  Meas/1 -> Subtract/2
  Switch/1 -> Add/1
  Constant7/1 -> Switch/1
  freeze/1 -> Switch/2
  Discrete-Time Integrator/1 -> Add1/2
  Add1/1 -> Sum2/2, Saturation/1
  Sum2/1 -> Kf/1
  Ord/1 -> Subtract/1, Add1/1
  Add/1 -> Discrete-Time Integrator/1
  Unit Delay/1 -> Add/2
  Saturation/1 -> Sum2/1, Out/1

== system sistema_polo_polo/VSC Controller Station 2/Discrete VSC Controller /Outer Active-Reactive Power and Voltage Loop/Active_Power_Control/Ramping ==
  note: Output is reset to zero when the ramp is not enabled
  note: Ramping
  enable_ramp : Inport
  Pref : Inport  Port=2
  Constant12 : Constant  Value=Ramp_apc
  Logical Operator7 : Logic  Operator=NOT  AllPortsSameDT=off
  Rate Limiter with external rates & reset (discrete) IC:0 : Subsystem  mask(Rate of Change Limiter){ic=0, st=Ts_Control}
      mask prompts: ic "Initial condition (pu):"; st "Sample time (s):"
      mask help: Limit rising and falling rates of signal. When the input (R) is true the output is reset to the input (In). Rates are in p.u./s for up and -p.u./s for down.
      mask Display: disp('                Rate\n               Limiter')
  Switch : Switch  Criteria=u2 > Threshold  SaturateOnIntegerOverflow=on
  zero : Constant  Value=0.0
  Pref_ramp : Outport
  wires:
  Logical Operator7/1 -> Rate Limiter with external rates & reset (discrete) IC:0/4(R)
  Switch/1 -> Rate Limiter with external rates & reset (discrete) IC:0/1(In)
  zero/1 -> Switch/3
  Pref/1 -> Switch/1
  enable_ramp/1 -> Logical Operator7/1, Switch/2
  Constant12/1 -> Rate Limiter with external rates & reset (discrete) IC:0/3(down_rate), Rate Limiter with external rates & reset (discrete) IC:0/2(up_rate)
  Rate Limiter with external rates & reset (discrete) IC:0/1(" ") -> Pref_ramp/1

== system sistema_polo_polo/VSC Controller Station 2/Discrete VSC Controller /Outer Active-Reactive Power and Voltage Loop/Current_Reference_Limitation/Double click here for  info ==
  note: Power System Simulation laboratory (IREQ)
  note: Current Reference Limitation
  note: The subsystem limits the amplitude of phase current of the fundamental component to the rated current
      | of the converter.
  note: Power Control Mode
  note: DC Voltage Control Mode
  note: In power control mode, equal scaling is applied to the active and reactive power reference when a limit is imposed.
  note: In DC voltage control mode, higher priority is given to the active power when a limit is imposed.

== system sistema_polo_polo/VSC Controller Station 2/Discrete VSC Controller /Outer Active-Reactive Power and Voltage Loop/DC_Voltage_Control/PI_regulator (type 2) ==
  note: Regulator PI
      | (Type 2)
  Ord : Inport
  Meas : Inport  Port=2
  Add : Sum
  Add1 : Sum
  Discrete-Time Integrator : DiscreteIntegrator  IntegratorMethod=Integration: Trapezoidal  gainval=Ki  InitialCondition=i_ic  SampleTime=Ts  LimitOutput=on  UpperSaturationLimit=max_i  LowerSaturationLimit=min_i  ICPrevOutput=DiscIntNeverNeededParam  ICPrevScaledInput=DiscIntNeverNeededParam
      settings: AttributesFormatString=Gain=%<gainval>\nMin=%<LowerSaturationLimit>\nMax=%<UpperSaturationLimit>
  Kf : Gain  Gain=Kf
      settings: AttributesFormatString=Gain=%<Gain>
  Kp : Gain  Gain=Kp
      settings: AttributesFormatString=Gain=%<Gain>
  Saturation : Saturate  UpperLimit=max_out  LowerLimit=min_out
      settings: AttributesFormatString=Min=%<LowerLimit>\nMax=%<UpperLimit>
  Subtract : Sum  Inputs=+-
  Sum2 : Sum  Inputs=|+-  SaturateOnIntegerOverflow=on
  Unit Delay : UnitDelay  SampleTime=Ts_Control
      settings: AttributesFormatString=IC=%<InitialCondition>
  Out : Outport
  wires:
  Kp/1 -> Add1/1
  Sum2/1 -> Kf/1
  Subtract/1 -> Add/1, Kp/1
  Saturation/1 -> Sum2/1, Out/1
  Unit Delay/1 -> Add/2
  Add/1 -> Discrete-Time Integrator/1
  Ord/1 -> Subtract/1
  Kf/1 -> Unit Delay/1
  Add1/1 -> Saturation/1, Sum2/2
  Discrete-Time Integrator/1 -> Add1/2
  Meas/1 -> Subtract/2

== system sistema_polo_polo/VSC Controller Station 2/Discrete VSC Controller /Outer Active-Reactive Power and Voltage Loop/Reactive_Power_Control/AC Voltage Control Override  ==
  note: Reset states when enabling
  note: Override Regulator
  note: Active when input (In) is outside its range [min_in, max_in] otherwise the output goes back to zero
  In : Inport
  Enable (reset) : EnablePort  StatesWhenEnabling=reset  PropagateVarSize=During execution
  Add : Sum
  Constant1 : Constant  Value=max_in
  Constant2 : Constant  Value=min_in
  Constant3 : Constant  Value=Kp
  Discrete-Time Integrator1 : DiscreteIntegrator  IntegratorMethod=Integration: Trapezoidal  gainval=Ki  InitialCondition=IC_i  SampleTime=Ts  LimitOutput=on  UpperSaturationLimit=0  LowerSaturationLimit=min_out_lim  ICPrevOutput=DiscIntNeverNeededParam  ICPrevScaledInput=DiscIntNeverNeededParam
      settings: AttributesFormatString=Gain=%<gainval>\nMin=%<LowerSaturationLimit>\nMax=%<UpperSaturationLimit>
  Discrete-Time Integrator2 : DiscreteIntegrator  IntegratorMethod=Integration: Trapezoidal  gainval=Ki  InitialCondition=IC_i  SampleTime=Ts  LimitOutput=on  UpperSaturationLimit=max_out_lim  LowerSaturationLimit=0  ICPrevOutput=DiscIntNeverNeededParam  ICPrevScaledInput=DiscIntNeverNeededParam
      settings: AttributesFormatString=Gain=%<gainval>\nMin=%<LowerSaturationLimit>\nMax=%<UpperSaturationLimit>
  Product : Product  RndMeth=Zero
  Saturation : Saturate  UpperLimit=0  LowerLimit=min_out_lim
      settings: AttributesFormatString=Min=%<LowerLimit>\nMax=%<UpperLimit>
  Saturation1 : Saturate  UpperLimit=max_out_lim  LowerLimit=0
      settings: AttributesFormatString=Min=%<LowerLimit>\nMax=%<UpperLimit>
  Saturation2 : Saturate  UpperLimit=max_out_lim  LowerLimit=min_out_lim
      settings: AttributesFormatString=Min=%<LowerLimit>\nMax=%<UpperLimit>
  Subtract : Sum  Inputs=+-
  Subtract1 : Sum  Inputs=-+
  Sum2 : Sum  Inputs=+++  SaturateOnIntegerOverflow=on
  Out : Outport
  wires:
  Constant2/1 -> Subtract1/2
  Constant1/1 -> Subtract/1
  Discrete-Time Integrator2/1 -> Sum2/3  "positive"
  Discrete-Time Integrator1/1 -> Sum2/2  "negative"
  Product/1 -> Sum2/1
  Saturation1/1 -> Add/2
  Saturation/1 -> Add/1
  Add/1 -> Product/2
  Constant3/1 -> Product/1
  In/1 -> Subtract1/1, Subtract/2
  Subtract/1 -> Discrete-Time Integrator1/1, Saturation/1
  Subtract1/1 -> Saturation1/1, Discrete-Time Integrator2/1
  Sum2/1 -> Saturation2/1
  Saturation2/1 -> Out/1

== system sistema_polo_polo/VSC Controller Station 2/Discrete VSC Controller /Outer Active-Reactive Power and Voltage Loop/Reactive_Power_Control/Freeze_integrator ==
  note: Freeze Integrator
  note: Low AC voltage level
  U_meas : Inport
  Constant8 : Constant  Value=V_level_rpc
  Relational Operator : RelationalOperator  Operator=<=
  Freeze : Outport
  wires:
  U_meas/1 -> Relational Operator/1
  Relational Operator/1 -> Freeze/1
  Constant8/1 -> Relational Operator/2

== system sistema_polo_polo/VSC Controller Station 2/Discrete VSC Controller /Outer Active-Reactive Power and Voltage Loop/Reactive_Power_Control/Int_regulator (type 1) ==
  note: Reset states when enabling
  note: Integral Regulator
      | (Type 1)
  Ord : Inport
  Meas : Inport  Port=2
  freeze : Inport  Port=3
  Enable (Reset) : EnablePort  StatesWhenEnabling=reset  PropagateVarSize=During execution
  Add : Sum
  Add1 : Sum
  Constant7 : Constant  Value=0.0
  Discrete-Time Integrator : DiscreteIntegrator  IntegratorMethod=Integration: Trapezoidal  gainval=Ki  InitialCondition=IC_i  SampleTime=Ts  LimitOutput=on  UpperSaturationLimit=max_i  LowerSaturationLimit=min_i  ICPrevOutput=DiscIntNeverNeededParam  ICPrevScaledInput=DiscIntNeverNeededParam
      settings: AttributesFormatString=Gain=%<gainval>\nMin=%<LowerSaturationLimit>\nMax=%<UpperSaturationLimit>
  Kf : Gain  Gain=Kf
      settings: AttributesFormatString=Gain=%<Gain>
  Saturation : Saturate  UpperLimit=max_out  LowerLimit=min_out
      settings: AttributesFormatString=Min=%<LowerLimit>\nMax=%<UpperLimit>
  Subtract : Sum  Inputs=+-
  Sum2 : Sum  Inputs=|+-  SaturateOnIntegerOverflow=on
  Switch : Switch  Criteria=u2 > Threshold  SaturateOnIntegerOverflow=on
  Unit Delay : UnitDelay  SampleTime=Ts_Control
      settings: AttributesFormatString=IC=%<InitialCondition>
  Out : Outport
  wires:
  Kf/1 -> Unit Delay/1
  Subtract/1 -> Switch/3
  Meas/1 -> Subtract/2
  Switch/1 -> Add/1
  Constant7/1 -> Switch/1
  freeze/1 -> Switch/2
  Discrete-Time Integrator/1 -> Add1/2
  Add1/1 -> Sum2/2, Saturation/1
  Sum2/1 -> Kf/1
  Ord/1 -> Subtract/1, Add1/1
  Add/1 -> Discrete-Time Integrator/1
  Unit Delay/1 -> Add/2
  Saturation/1 -> Sum2/1, Out/1

== system sistema_polo_polo/VSC Controller Station 1/Discrete VSC Controller /Outer Active-Reactive Power and Voltage Loop/Active_Power_Control/Ramping/Rate Limiter with external rates & reset (discrete) IC:0 ==
  note: Rate Limiter with external rates & reset (Discrete)
  note: IC=ic
  note: Max= 4
      | Min =1
  note: Silvano Casoria
      | IREQ
  In : Inport
  up_rate : Inport  Port=2
  down_rate : Inport  Port=3
  R : Inport  Port=4
  Abs : Abs  SaturateOnIntegerOverflow=on
  Constant3 : Constant
  Data Type Conversion1 : DataTypeConversion  SaturateOnIntegerOverflow=on  RndMeth=Zero
  Data Type Conversion2 : DataTypeConversion  SaturateOnIntegerOverflow=on  RndMeth=Zero
  Data Type Conversion3 : DataTypeConversion  SaturateOnIntegerOverflow=on  RndMeth=Zero
  Gain1 : Gain  Gain=2  SaturateOnIntegerOverflow=on  OutDataTypeStr=Inherit: Same as input  ParamDataTypeStr=Inherit: Same as input
  Gain2 : Gain  Gain=3  SaturateOnIntegerOverflow=on  OutDataTypeStr=Inherit: Same as input  ParamDataTypeStr=Inherit: Same as input
  Gain3 : Gain  Gain=st  SaturateOnIntegerOverflow=on  OutDataTypeStr=Inherit: Same as input  ParamDataTypeStr=Inherit: Same as input
  Gain4 : Gain  Gain=-st  SaturateOnIntegerOverflow=on  OutDataTypeStr=Inherit: Same as input  ParamDataTypeStr=Inherit: Same as input
  Multiport Switch : MultiPortSwitch  Inputs=4  SaturateOnIntegerOverflow=on  InputSameDT=on
  Relational Operator : RelationalOperator  Operator=>  InputSameDT=on
  Relational Operator2 : RelationalOperator  Operator=<  InputSameDT=on
  Saturation : Saturate  UpperLimit=4  LowerLimit=1
  Sum : Sum  Inputs=+-  SaturateOnIntegerOverflow=on  InputSameDT=on  OutDataTypeStr=Inherit: Same as first input
  Sum1 : Sum  Inputs=++++  SaturateOnIntegerOverflow=on  InputSameDT=on  OutDataTypeStr=Inherit: Same as first input
  Sum2 : Sum  SaturateOnIntegerOverflow=on  InputSameDT=on  OutDataTypeStr=Inherit: Same as first input
  Sum3 : Sum  SaturateOnIntegerOverflow=on  InputSameDT=on  OutDataTypeStr=Inherit: Same as first input
  Unit Delay : UnitDelay  InitialCondition=ic  SampleTime=st
  " " : Outport  InitialOutput=0
  wires:
  Gain2/1 -> Sum1/3
  Constant3/1 -> Sum1/4
  Relational Operator/1 -> Data Type Conversion2/1
  Gain1/1 -> Sum1/2
  Saturation/1 -> Multiport Switch/1
  Sum1/1 -> Saturation/1
  R/1 -> Data Type Conversion3/1
  Sum3/1 -> Multiport Switch/4
  Sum2/1 -> Multiport Switch/3
  In/1 -> Multiport Switch/5, Multiport Switch/2, Sum/1
  Relational Operator2/1 -> Data Type Conversion1/1
  Sum/1 -> Relational Operator2/1, Relational Operator/1  "Rate"
  Multiport Switch/1 -> " "/1, Unit Delay/1
  Gain4/1 -> Sum3/2, Relational Operator2/2
  Gain3/1 -> Sum2/2, Relational Operator/2
  Unit Delay/1 -> Sum3/1, Sum2/1, Sum/2
  up_rate/1 -> Gain3/1
  down_rate/1 -> Abs/1
  Abs/1 -> Gain4/1
  Data Type Conversion1/1 -> Gain1/1
  Data Type Conversion2/1 -> Sum1/1
  Data Type Conversion3/1 -> Gain2/1

== system sistema_polo_polo/VSC Controller Station 2/Discrete VSC Controller /Outer Active-Reactive Power and Voltage Loop/Active_Power_Control/Ramping/Rate Limiter with external rates & reset (discrete) IC:0 ==
  note: Rate Limiter with external rates & reset (Discrete)
  note: IC=ic
  note: Max= 4
      | Min =1
  note: Silvano Casoria
      | IREQ
  In : Inport
  up_rate : Inport  Port=2
  down_rate : Inport  Port=3
  R : Inport  Port=4
  Abs : Abs  SaturateOnIntegerOverflow=on
  Constant3 : Constant
  Data Type Conversion1 : DataTypeConversion  SaturateOnIntegerOverflow=on  RndMeth=Zero
  Data Type Conversion2 : DataTypeConversion  SaturateOnIntegerOverflow=on  RndMeth=Zero
  Data Type Conversion3 : DataTypeConversion  SaturateOnIntegerOverflow=on  RndMeth=Zero
  Gain1 : Gain  Gain=2  SaturateOnIntegerOverflow=on  OutDataTypeStr=Inherit: Same as input  ParamDataTypeStr=Inherit: Same as input
  Gain2 : Gain  Gain=3  SaturateOnIntegerOverflow=on  OutDataTypeStr=Inherit: Same as input  ParamDataTypeStr=Inherit: Same as input
  Gain3 : Gain  Gain=st  SaturateOnIntegerOverflow=on  OutDataTypeStr=Inherit: Same as input  ParamDataTypeStr=Inherit: Same as input
  Gain4 : Gain  Gain=-st  SaturateOnIntegerOverflow=on  OutDataTypeStr=Inherit: Same as input  ParamDataTypeStr=Inherit: Same as input
  Multiport Switch : MultiPortSwitch  Inputs=4  SaturateOnIntegerOverflow=on  InputSameDT=on
  Relational Operator : RelationalOperator  Operator=>  InputSameDT=on
  Relational Operator2 : RelationalOperator  Operator=<  InputSameDT=on
  Saturation : Saturate  UpperLimit=4  LowerLimit=1
  Sum : Sum  Inputs=+-  SaturateOnIntegerOverflow=on  InputSameDT=on  OutDataTypeStr=Inherit: Same as first input
  Sum1 : Sum  Inputs=++++  SaturateOnIntegerOverflow=on  InputSameDT=on  OutDataTypeStr=Inherit: Same as first input
  Sum2 : Sum  SaturateOnIntegerOverflow=on  InputSameDT=on  OutDataTypeStr=Inherit: Same as first input
  Sum3 : Sum  SaturateOnIntegerOverflow=on  InputSameDT=on  OutDataTypeStr=Inherit: Same as first input
  Unit Delay : UnitDelay  InitialCondition=ic  SampleTime=st
  " " : Outport  InitialOutput=0
  wires:
  Gain2/1 -> Sum1/3
  Constant3/1 -> Sum1/4
  Relational Operator/1 -> Data Type Conversion2/1
  Gain1/1 -> Sum1/2
  Saturation/1 -> Multiport Switch/1
  Sum1/1 -> Saturation/1
  R/1 -> Data Type Conversion3/1
  Sum3/1 -> Multiport Switch/4
  Sum2/1 -> Multiport Switch/3
  In/1 -> Multiport Switch/5, Multiport Switch/2, Sum/1
  Relational Operator2/1 -> Data Type Conversion1/1
  Sum/1 -> Relational Operator2/1, Relational Operator/1  "Rate"
  Multiport Switch/1 -> " "/1, Unit Delay/1
  Gain4/1 -> Sum3/2, Relational Operator2/2
  Gain3/1 -> Sum2/2, Relational Operator/2
  Unit Delay/1 -> Sum3/1, Sum2/1, Sum/2
  up_rate/1 -> Gain3/1
  down_rate/1 -> Abs/1
  Abs/1 -> Gain4/1
  Data Type Conversion1/1 -> Gain1/1
  Data Type Conversion2/1 -> Sum1/1
  Data Type Conversion3/1 -> Gain2/1
